simulink model "kalmanfilter"  (Simulink 10.3)
settings: Solver=FixedStepDiscrete  StartTime=0.0  StopTime=10.0  RelTol=1e-3  EnableMultiTasking=on
values from neighbouring files (symbols this model uses):
  F = [0.8110   -0.0348    0.0499    0.3313 ... (first row only)    [runkalmanfilter.m]
  F1 = F + 0*randn(size(F))    [runkalmanfilter.m]
  G = [-0.0130    0.0024 ... (first row only)    [runkalmanfilter.m]
  G1 = G + 0*randn(size(G))    [runkalmanfilter.m]
  H = [0.1685   -0.9595   -0.0755   -0.3771 ... (first row only)    [runkalmanfilter.m]    (also in runllmse.m = randn(N,4))
  H1 = H + p*randn(size(H))    [runkalmanfilter.m]
  P1 = 0*eye(4,4)    [runkalmanfilter.m]
  Q = diag([0.8^2 0.5^2])    [runkalmanfilter.m]
  Q1 = Q    [runkalmanfilter.m]
  R = .1*eye(2)    [runkalmanfilter.m]
  R1 = R    [runkalmanfilter.m]
  x0 = 4*randn(4,1)    [runkalmanfilter.m]
  x1 = x0    [runkalmanfilter.m]
libraries: dspinverses x1, dspmtrx3 x1
settings Model: Creator=fo1521  LastModifiedBy=j21lys
settings DataIOCC: LimitDataPoints=on
settings OptimizationCC: InitFltsAndDblsToZero=on
settings DebuggingCC: SaveWithParameterizedLinksMsg=none  SolverPrmCheckMsg=warning  MultiTaskCondExecSysMsg=none
settings HardwareCC: TargetHWDeviceType=32-bit Generic
settings GRTTargetCC: TargetFcnLib=ansi_tfl_tmw.mat

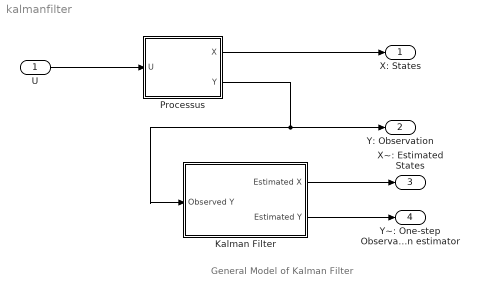
== system kalmanfilter ==
  note: General Model of Kalman Filter
  U : Inport  PortDimensions=size(G,2)
  Kalman Filter : Subsystem
  "Processus " : Subsystem
  X: States : Outport
  Y: Observation : Outport  Port=2
  X~: Estimated States : Outport  Port=3
  Y~: One-step Observation estimator : Outport  Port=4
  wires:
  "Processus "/2(Y) -> Kalman Filter/1(Observed Y), Y: Observation/1
  "Processus "/1(X) -> X: States/1
  Kalman Filter/1(Estimated X) -> X~: Estimated States/1
  Kalman Filter/2(Estimated Y) -> Y~: One-step Observation estimator/1
  U/1 -> "Processus "/1(U)

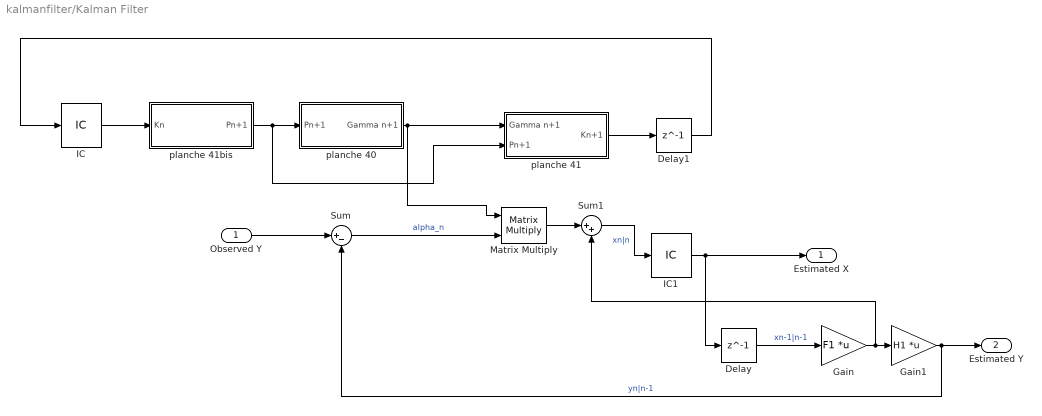
== system kalmanfilter/Kalman Filter ==
  Observed Y : Inport  PortDimensions=size(H,1)
  Delay : Delay  DelayLength=1  InitialCondition=0
  Delay1 : Delay  DelayLength=1  InitialCondition=0
  Gain : Gain  Gain=F1  Multiplication=Matrix(K*u)
  Gain1 : Gain  Gain=H1  Multiplication=Matrix(K*u)
  IC : InitialCondition  Value=P1
  IC1 : InitialCondition  Value=x1
  Matrix Multiply : Product  Multiplication=Matrix(*)
  Sum : Sum  Inputs=|+-
  Sum1 : Sum  Inputs=|++
  planche 40 : Subsystem
  planche 41 : Subsystem
  planche 41bis : Subsystem
  Estimated X : Outport
  Estimated Y : Outport  Port=2
  wires:
  Observed Y/1 -> Sum/1
  Delay/1 -> Gain/1  "xn-1|n-1"
  Sum/1 -> Matrix Multiply/2  "alpha_n"
  Gain/1 -> Sum1/2, Gain1/1
  Gain1/1 -> Sum/2, Estimated Y/1  "yn|n-1"
  Matrix Multiply/1 -> Sum1/1
  Sum1/1 -> IC1/1  "xn|n"
  IC1/1 -> Delay/1, Estimated X/1
  IC/1 -> planche 41bis/1(Kn)
  planche 41bis/1(Pn+1) -> planche 41/2(Pn+1), planche 40/1(Pn+1)
  planche 41/1(Kn+1) -> Delay1/1
  Delay1/1 -> IC/1
  planche 40/1(Gamma n+1) -> Matrix Multiply/1, planche 41/1(Gamma n+1)

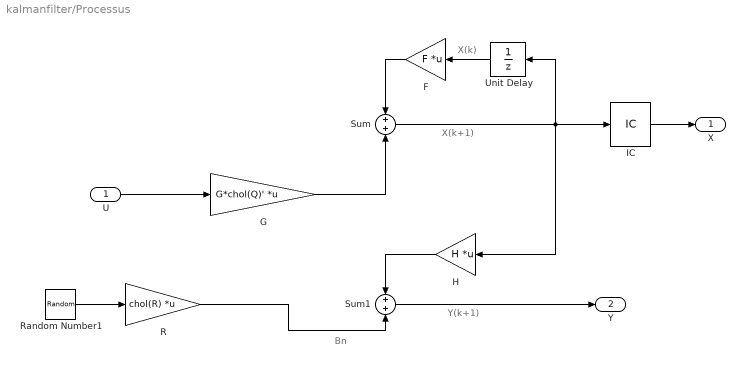
== system kalmanfilter/Processus  ==
  note: X(k+1)
  note: Y(k+1)
  note: X(k)
  note: Bn
  U : Inport  PortDimensions=size(G,2)
  F : Gain  Gain=F  Multiplication=Matrix(K*u)
  G : Gain  Gain=G*chol(Q)'  Multiplication=Matrix(K*u)
  H : Gain  Gain=H  Multiplication=Matrix(K*u)
  IC : InitialCondition  Value=x0
  R : Gain  Gain=chol(R)  Multiplication=Matrix(K*u)
  Random Number1 : RandomNumber  Mean=zeros(size(R,1),1)  Variance=ones(size(R,1),1)  SampleTime=1
  Sum : Sum
  Sum1 : Sum
  Unit Delay : UnitDelay
  X : Outport
  Y : Outport  Port=2
  wires:
  H/1 -> Sum1/1
  Random Number1/1 -> R/1
  Sum1/1 -> Y/1
  Sum/1 -> IC/1, Unit Delay/1, H/1
  Unit Delay/1 -> F/1
  F/1 -> Sum/1
  G/1 -> Sum/2
  R/1 -> Sum1/2
  U/1 -> G/1
  IC/1 -> X/1

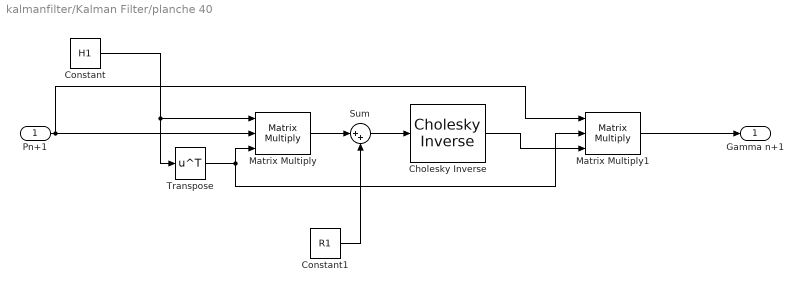
== system kalmanfilter/Kalman Filter/planche 40 ==
  Pn+1 : Inport
  Cholesky Inverse : dspinverses/Cholesky Inverse  errmode=Warning
      settings: SourceProductBaseCode=DS
  Constant : Constant  Value=H1
  Constant1 : Constant  Value=R1
  Matrix Multiply : Product  Inputs=3  Multiplication=Matrix(*)
  Matrix Multiply1 : Product  Inputs=3  Multiplication=Matrix(*)
  Sum : Sum  Inputs=|++
  Transpose : Math  Operator=transpose  SaturateOnIntegerOverflow=on
  Gamma n+1 : Outport
  wires:
  Pn+1/1 -> Matrix Multiply1/1, Matrix Multiply/2
  Constant/1 -> Transpose/1, Matrix Multiply/1
  Transpose/1 -> Matrix Multiply1/2, Matrix Multiply/3
  Matrix Multiply/1 -> Sum/1
  Constant1/1 -> Sum/2
  Matrix Multiply1/1 -> Gamma n+1/1
  Sum/1 -> Cholesky Inverse/1
  Cholesky Inverse/1 -> Matrix Multiply1/3

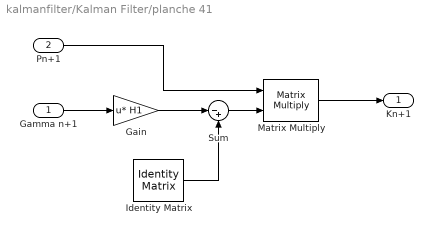
== system kalmanfilter/Kalman Filter/planche 41 ==
  Gamma n+1 : Inport
  Pn+1 : Inport  Port=2
  Gain : Gain  Gain=H1  Multiplication=Matrix(u*K)
  Identity Matrix : dspmtrx3/Identity Matrix  Inherit=off  N=4  Ts=1  dataType=double  isSigned=on  wordLen=16  udDataType=sfix(16)  fracBitsMode=Best precision  numFracBits=15  OutDataTypeStr=double  LastOutDataTypeStr=double
  Matrix Multiply : Product  Multiplication=Matrix(*)
  Sum : Sum  Inputs=|-+
  Kn+1 : Outport
  wires:
  Gamma n+1/1 -> Gain/1
  Gain/1 -> Sum/1
  Identity Matrix/1 -> Sum/2
  Sum/1 -> Matrix Multiply/2
  Pn+1/1 -> Matrix Multiply/1
  Matrix Multiply/1 -> Kn+1/1

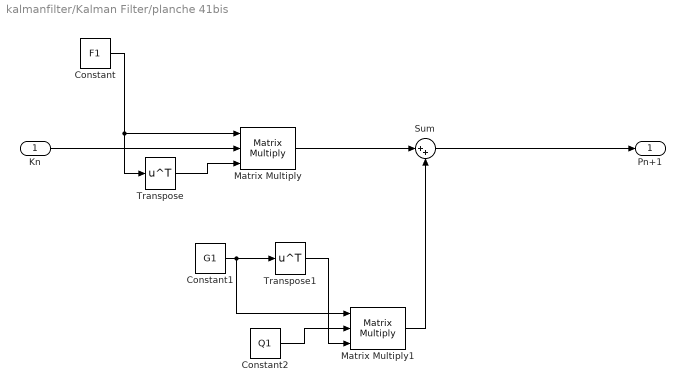
== system kalmanfilter/Kalman Filter/planche 41bis ==
  Kn : Inport
  Constant : Constant  Value=F1
  Constant1 : Constant  Value=G1
  Constant2 : Constant  Value=Q1
  Matrix Multiply : Product  Inputs=3  Multiplication=Matrix(*)
  Matrix Multiply1 : Product  Inputs=3  Multiplication=Matrix(*)
  Sum : Sum  Inputs=|++
  Transpose : Math  Operator=transpose  SaturateOnIntegerOverflow=on
  Transpose1 : Math  Operator=transpose  SaturateOnIntegerOverflow=on
  Pn+1 : Outport
  wires:
  Constant/1 -> Matrix Multiply/1, Transpose/1
  Transpose/1 -> Matrix Multiply/3
  Constant1/1 -> Matrix Multiply1/1, Transpose1/1
  Kn/1 -> Matrix Multiply/2
  Transpose1/1 -> Matrix Multiply1/3
  Constant2/1 -> Matrix Multiply1/2
  Matrix Multiply/1 -> Sum/1
  Matrix Multiply1/1 -> Sum/2
  Sum/1 -> Pn+1/1
